simulink model "calcEnergieAndMagneticField"  (R2016a)
settings: Solver=FixedStepDiscrete  StartTime=0.0  StopTime=3600  FixedStep=1  RelTol=1e-3
libraries: simulink x1
settings Model: Creator=franz  LastModifiedBy=franz
settings SolverCC: AutoInsertRateTranBlk=on
settings DataIOCC: SaveOutput=off  SaveTime=off
settings OptimizationCC: DefaultParameterBehavior=Inlined  InlineInvariantSignals=on  StateBitsets=on  DataBitsets=on  ZeroExternalMemoryAtStartup=off  ZeroInternalMemoryAtStartup=off  NoFixptDivByZeroProtection=on  OptimizeModelRefInitCode=on  LifeSpan=1
settings HardwareCC: ProdBitPerPointer=32  ProdLargestAtomicFloat=None  ProdIntDivRoundTo=Floor  ProdWordSize=32  ProdHWDeviceType=Generic->Custom
settings RTWCC: SystemTargetFile=ert.tlc  TLCOptions=-p0  GenCodeOnly=on  TemplateMakefile=ert_default_tmf  GenerateReport=on  RTWVerbose=off  IncludeHyperlinkInReport=on  LaunchReport=on  GenerateTraceInfo=on  GenerateTraceReport=on  GenerateTraceReportSl=on  GenerateTraceReportSf=on  GenerateTraceReportEml=on
settings CodeAppCC: ForceParamTrailComments=on  IgnoreCustomStorageClasses=off  OperatorAnnotations=on  SimulinkDataObjDesc=on  SFDataObjDesc=on  MATLABFcnDesc=on  CustomSymbolStrGlobalVar=rt$N$M  CustomSymbolStrType=$N$M  CustomSymbolStrFcn=$N$M$F  CustomSymbolStrMacro=$N$M  InsertBlockDesc=on  MATLABSourceComments=on
settings ERTTargetCC: CodeReplacementLibrary=ISO_C  GenerateSampleERTMain=on  IncludeMdlTerminateFcn=off  SuppressErrorStatus=on  SupportAbsoluteTime=off  SupportNonFinite=off  SupportComplex=off  PurelyIntegerCode=on  InlinedParameterPlacement=NonHierarchical  RootIOFormat=Structure reference  ERTCustomFileTemplate=example_file_process.tlc

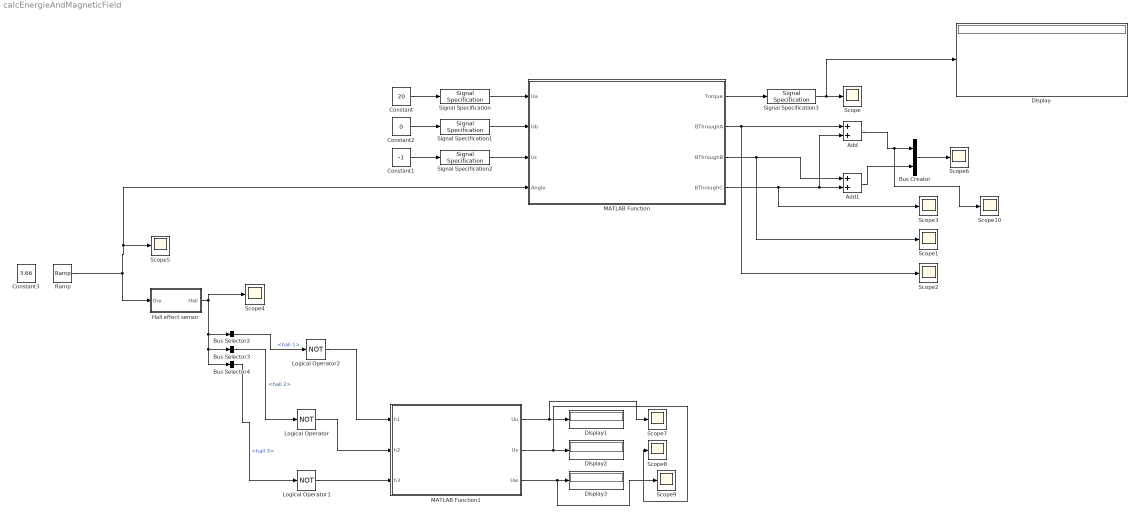
== system calcEnergieAndMagneticField ==
  Add : Sum
  Add1 : Sum
  Bus Creator : BusCreator  Inputs=2
  Bus Selector2 : BusSelector  OutputSignals=hall 1
  Bus Selector3 : BusSelector  OutputSignals=hall 2
  Bus Selector4 : BusSelector  OutputSignals=hall 3
  Constant : Constant  Value=20
  Constant1 : Constant  Value=-1
  Constant2 : Constant  Value=0
  Constant3 : Constant  Value=3.66
  Display{,1..3} (4 alike) : Display
  Hall effect sensor : Subsystem  AncestorBlock=spsPMSynchronousMachineModel/Continuous/Hall effect sensor
  Logical Operator : Logic  Operator=NOT  AllPortsSameDT=off  OutDataTypeStr=boolean
  Logical Operator1 : Logic  Operator=NOT  AllPortsSameDT=off  OutDataTypeStr=boolean
  Logical Operator2 : Logic  Operator=NOT  AllPortsSameDT=off  OutDataTypeStr=boolean
  MATLAB Function : MATLAB Function  TreatAsAtomicUnit=on
  MATLAB Function1 : MATLAB Function  TreatAsAtomicUnit=on
  Ramp : simulink/Sources/Ramp  slope=0.05  start=0  X0=0
  Scope{,1..10} (11 alike) : Scope
  Signal Specification : SignalSpecification  Unit=V
  Signal Specification1 : SignalSpecification  Unit=V
  Signal Specification2 : SignalSpecification  Unit=V
  Signal Specification3 : SignalSpecification  Unit=Nm
  wires:
  MATLAB Function1/1(Uu) -> Scope7/1, Display1/1
  MATLAB Function1/2(Uv) -> Scope8/1, Display2/1
  MATLAB Function/1(Torque) -> Signal Specification3/1
  Signal Specification/1 -> MATLAB Function/1(Ua)
  Signal Specification2/1 -> MATLAB Function/3(Uc)
  Signal Specification1/1 -> MATLAB Function/2(Ub)
  MATLAB Function/4(BThroughC) -> Scope3/1, Add1/2, Add/2
  MATLAB Function/2(BThroughA) -> Scope2/1, Add/1
  Signal Specification3/1 -> Display/1, Scope/1
  Hall effect sensor/1(Hall) -> Scope4/1, Bus Selector4/1, Bus Selector3/1, Bus Selector2/1
  Bus Creator/1 -> Scope6/1
  Add/1 -> Scope10/1, Bus Creator/1
  Add1/1 -> Bus Creator/2
  Ramp/1 -> Scope5/1, MATLAB Function/4(Angle), Hall effect sensor/1(the)
  MATLAB Function/3(BThroughB) -> Scope1/1, Add1/1
  Bus Selector2/1 -> Logical Operator2/1  "<hall 1>"
  Logical Operator2/1 -> MATLAB Function1/1(h1)
  Bus Selector3/1 -> Logical Operator/1  "<hall 2>"
  Logical Operator/1 -> MATLAB Function1/2(h2)
  Bus Selector4/1 -> Logical Operator1/1  "<hall 3>"
  Logical Operator1/1 -> MATLAB Function1/3(h3)
  MATLAB Function1/3(Uw) -> Scope9/1, Display3/1
  Constant/1 -> Signal Specification/1
  Constant2/1 -> Signal Specification1/1
  Constant1/1 -> Signal Specification2/1

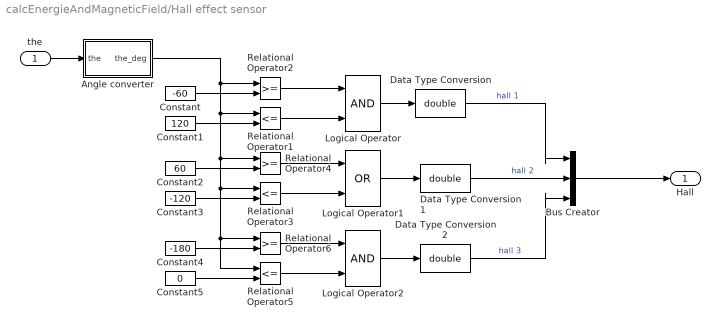
== system calcEnergieAndMagneticField/Hall effect sensor ==
  the : Inport
  Angle converter : Subsystem
  Bus Creator : BusCreator  Inputs=3
  Constant : Constant  Value=-60
  Constant1 : Constant  Value=120
  Constant2 : Constant  Value=60
  Constant3 : Constant  Value=-120
  Constant4 : Constant  Value=-180
  Constant5 : Constant  Value=0
  Data Type Conversion : DataTypeConversion  OutDataTypeStr=double  SaturateOnIntegerOverflow=on  RndMeth=Zero
  Data Type Conversion1 : DataTypeConversion  OutDataTypeStr=double  SaturateOnIntegerOverflow=on  RndMeth=Zero
  Data Type Conversion2 : DataTypeConversion  OutDataTypeStr=double  SaturateOnIntegerOverflow=on  RndMeth=Zero
  Logical Operator : Logic  AllPortsSameDT=off  OutDataTypeStr=boolean
  Logical Operator1 : Logic  Operator=OR  AllPortsSameDT=off  OutDataTypeStr=boolean
  Logical Operator2 : Logic  AllPortsSameDT=off  OutDataTypeStr=boolean
  Relational Operator1 : RelationalOperator  Operator=<=  InputSameDT=on
  Relational Operator2 : RelationalOperator  InputSameDT=on
  Relational Operator3 : RelationalOperator  Operator=<=  InputSameDT=on
  Relational Operator4 : RelationalOperator  InputSameDT=on
  Relational Operator5 : RelationalOperator  Operator=<=  InputSameDT=on
  Relational Operator6 : RelationalOperator  InputSameDT=on
  Hall : Outport
  wires:
  Bus Creator/1 -> Hall/1
  Data Type Conversion2/1 -> Bus Creator/3  "hall 3"
  Data Type Conversion1/1 -> Bus Creator/2  "hall 2"
  Data Type Conversion/1 -> Bus Creator/1  "hall 1"
  Relational Operator5/1 -> Logical Operator2/2
  Logical Operator2/1 -> Data Type Conversion2/1
  Relational Operator6/1 -> Logical Operator2/1
  Constant4/1 -> Relational Operator6/2
  Constant5/1 -> Relational Operator5/2
  Relational Operator3/1 -> Logical Operator1/2
  Logical Operator1/1 -> Data Type Conversion1/1
  Logical Operator/1 -> Data Type Conversion/1
  Relational Operator2/1 -> Logical Operator/1
  Relational Operator1/1 -> Logical Operator/2
  Angle converter/1(the_deg) -> Relational Operator2/1, Relational Operator1/1, Relational Operator6/1, Relational Operator5/1, Relational Operator3/1, Relational Operator4/1
  Constant/1 -> Relational Operator2/2
  Constant1/1 -> Relational Operator1/2
  Relational Operator4/1 -> Logical Operator1/1
  Constant2/1 -> Relational Operator4/2
  Constant3/1 -> Relational Operator3/2
  the/1 -> Angle converter/1(the)

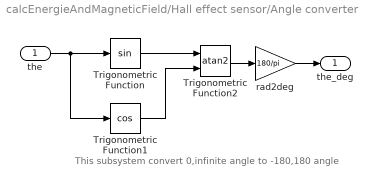
== system calcEnergieAndMagneticField/Hall effect sensor/Angle converter ==
  note: This subsystem convert 0,infinite angle to -180,180 angle
  the : Inport
  Trigonometric Function : Trigonometry
  Trigonometric Function1 : Trigonometry  Operator=cos
  Trigonometric Function2 : Trigonometry  Operator=atan2
  rad2deg : Gain  Gain=180/pi  SaturateOnIntegerOverflow=on  OutDataTypeStr=Inherit: Same as input  ParamDataTypeStr=Inherit: Same as input
  the_deg : Outport
  wires:
  the/1 -> Trigonometric Function/1, Trigonometric Function1/1
  Trigonometric Function/1 -> Trigonometric Function2/1
  Trigonometric Function1/1 -> Trigonometric Function2/2
  Trigonometric Function2/1 -> rad2deg/1
  rad2deg/1 -> the_deg/1

== matlab function calcEnergieAndMagneticField/MATLAB Function1 ==
  data: h1 input; Uu output; h2 input; h3 input; Uv output; Uw output
function [Uu, Uv, Uw] = HBridge(h1, h2, h3)

key = h1*4+h2+2*h3;

    Uu = -1;
    Uv = -1;
    Uw = -1;

switch key
  case 2
    Uu = 20;
    Uv = 0;
    Uw = -1;
  case 6
    Uu = -1;
    Uv = 0;
    Uw = 20;
  case 4
    Uu = 0;
    Uv = -1;
    Uw = 20;
  case 5
    Uu = 0;
    Uv = 20;
    Uw = -1;    
  case 1
    Uu = -1;
    Uv = 20;
    Uw = 0;
  case 3
    Uu = 20;
    Uv = -1;
    Uw = 0;
end

== matlab function calcEnergieAndMagneticField/MATLAB Function ==
  data: Ua input; Torque output; Ub input; Uc input; Angle input; BThroughA output; BThroughB output; BThroughC output
function [ Torque, BThroughA, BThroughB, BThroughC ] = calcEnergyAndMagneticField( Ua, Ub, Uc, Angle )
       
    %constant
    u0 = 4*pi*10^(-7);   % H/m
    multiplier = 7*20;
    
    %variables that have to be specified
    coilResistence = 0.33; %Ohm resistance of 2 coils in a row
    coilConstant = 42; %u0*(12/(28*10^(-3))); %u0*(n/l)    n=12 pro zahn (4 Zähne pro Spule), l= länge in (dstator - dshaft = 34 -6=) 28mm, μ0 = 4π·10−7 H/m, im zwischen raum befindet sich luft, somit kann µr vernachlässigt werden
    bRotor = 0.42;  %flussdichte des festen magnetfeldes

    %all magnetic field variants
    nStator = ones(1, 7*multiplier);
    sStator = (-1)*nStator;
    fieldLess = 0*nStator;
    
    case1 = [sStator, nStator, sStator, nStator, sStator, nStator, sStator, nStator, fieldLess, fieldLess, fieldLess, fieldLess];
    case2 = (-1)*case1;
    case3 = [sStator, nStator, sStator, nStator, fieldLess, fieldLess, fieldLess, fieldLess, nStator, sStator, nStator, sStator];
    case4 = (-1)*case3;
    case5 = [fieldLess, fieldLess, fieldLess, fieldLess, sStator, nStator, sStator, nStator, sStator, nStator, sStator, nStator];
    case6 = (-1)*case5;
    
    %determine which kind of current feed ist applyed
    voltage = 0;
    currentCase = zeros(1, 84*multiplier);
    if Ua==0
        if (Ub>0 && Uc<0)
            voltage = Ub;
            currentCase = case2;
        elseif (Ub<0 && Uc>0)
            voltage = Uc;
            currentCase = case4;            
        end
        
    elseif Ub==0
        if (Ua>0 && Uc<0)
            voltage = Ua;
            currentCase = case1;
        elseif (Ua<0 && Uc>0)
            voltage = Uc;
            currentCase = case5;            
        end
        
    elseif Uc==0
        if (Ua>0 && Ub<0)
            voltage = Ua;
            currentCase = case3;
        elseif (Ua<0 && Ub>0)
            voltage = Ub;
            currentCase = case6;            
        end
    end

    
    %fill rotor magnetic-flow field
    rotor = zeros(1, 84*multiplier);
    sign = 1;
    for i=1:84*multiplier
        rotor(i) = sign*bRotor;
        if mod(i, 6*multiplier)==0
            sign = sign*(-1);
        end
    end
            
    %rotatet rotor field 
    startOffset = mod(round(Angle/(360/(84*multiplier))), 84*multiplier)+1;
    rotor = [rotor(startOffset:length(rotor)), rotor(1:startOffset-1)];
    %rotate one step more, needed later for calculation of delta W
    rotorP1 =[rotor(length(rotor)), rotor(1:(length(rotor)-1))];

    %current
    I = voltage/coilResistence;
    
    %fild pro Coil without sign
    hCoil = coilConstant*I;
    
    %field from stator with correct signs
    BSTATOR = (ones(1, 84*multiplier) * hCoil).*currentCase;
   
    %resulting magnetic flow
    Bres = BSTATOR+rotor;
    Bresp1 = BSTATOR+rotorP1;
    
    Wres = (Bres.^2)/(2*u0);
    Wresp1 = (Bresp1.^2)/(2*u0);
    
    deltaW = sum(Wres)-sum(Wresp1);
    
    %because we asume that delta x is 84/360*2*pi*r and we want to get M
    %(which is F*r)
    %later we can divide deltaW by (360*2*pi) and get M
    Torque = deltaW/(360*2*pi);
    
    
    %identify magnetic field through coil
    BThroughATemp = Bres(1:28*multiplier);
    BThroughBTemp = Bres(1+1*28*multiplier:2*28*multiplier);
    BThroughCTemp = Bres(1+2*28*multiplier:3*28*multiplier);
    
    %output magneticfield over coil
    BThroughA = sum(BThroughATemp);
    BThroughB = sum(BThroughBTemp);
    BThroughC = sum(BThroughCTemp);
end
